simulink model "two_tanks_baseline"  (Simulink 7.3)
settings: Solver=ode45  StartTime=0.0  StopTime=1000  MaxStep=.01  RelTol=1e-3
model workspace (MAT data in the model file):
  x1o : Simulink.Parameter (value not decoded)
  a1 : Simulink.Parameter (value not decoded)
  a2 : Simulink.Parameter (value not decoded)
  A_1 : Simulink.Parameter (value not decoded)
  A_2 : Simulink.Parameter (value not decoded)
  gamma : Simulink.Parameter (value not decoded)
  g : Simulink.Parameter (value not decoded)
  x1_max : Simulink.Parameter (value not decoded)
  x2_max : Simulink.Parameter (value not decoded)
  u_max : Simulink.Parameter (value not decoded)
settings Model: Creator=Administrator  LastModifiedBy=Administrator

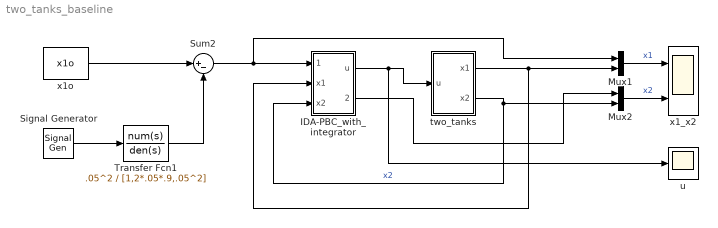
== system two_tanks_baseline ==
  IDA-PBC_with_integrator : Subsystem  mask{eps2=4, eps3=.75, q=10, A_1=A_1, A_2=A_2, a1=a1, a2=a2, gamma=gamma, u_max=u_max, x1_max=x1_max, g=g}
      mask prompts: eps2 "eps2 > 1"; eps3 "0 < eps3 < 1"; q "q > 0"; A_1 "A_1 (cm^2)"; A_2 "A_2 (cm^2)"; a1 "a1 (cm^2)"; a2 "a2 (cm^2)"; g "g (cm/s^2)"
      mask init:
      | k1 = 1;
      | if eps2 <= 1
      |     eps2 = 1.01;
      | end
      | k2 = eps2*A_2 / (4*A_1) ;
      | if eps3 >= 1
      |     eps3 = 0.99;
      | end
      | k3 = eps3*((4*k2*A_1-A_2)/(k2*A_1^2));
      | E_Qd=eig([-1/(k1*A_1),1/(k2*A_1),0;0,-1/(k2*A_2),0;k3/k1,0,-k3/k1])
      | p = [k1;-k2*gamma+k1*k2*k3-k2*k3+k2;k1^2]
      | cl_num = k2^2*gamma^2 + ((1-k1)*k2^2*k3 - 2*k2^2)*gamma + (k1-1)*k2^2*k3 + k2^2 + k1^3 + k1^2;
      | cl_den = k2^2*gamma^2 + 2*((1-k1)*k3-1)*k2^2*gamma + (k1^2-2*k1+1)*k2^2*k3^2 + 2*(k1-1)*k2^2*k3 + k2^2 + k1^4 + k1^2;
      | cl = -cl_num/cl_den
  Mux1 : Mux  Inputs=2
  Mux2 : Mux  Inputs=2
  Signal Generator : SignalGenerator  WaveForm=square  Amplitude=.95*x1o  Frequency=1/1000
  Sum2 : Sum  Inputs=|+-  OutDataType=fixdt(1, 16)  OutScaling=2^0
  Transfer Fcn1 : TransferFcn  Numerator=.05^2  Denominator=[1,2*.05*.9,.05^2]
  two_tanks : Subsystem  mask{x1o=x1o, x2o=x1o*((1-gamma)*a1/a2)^2, a1=a1, a2=a2, A_1=A_1, A_2=A_2, gamma=gamma, u_max=u_max, x1_max=x1_max, x2_max=x2_max, g=g, ku=1}
      mask prompts: x1o "x1o (cm)"; x2o "x2o (cm)"; a1 "a1 (cm2)"; a2 "a2 (cm2)"; A_1 "A_1 (cm2)"; A_2 "A_2 (cm2)"; gamma "gamma in [0,1]"; g "g (cm/s2)"
  u : Scope
      settings: YMin=5  YMax=70  SaveName=ScopeData2  SampleInput=on  SampleTime=.5
  x1_x2 : Scope  NumInputPorts=2
      settings: YMin=0~0  YMax=40~80  SampleInput=on  SampleTime=.5
  x1o : Constant  Value=x1o  OutDataType=fixdt(1, 16)  OutScaling=2^0
  wires:
  x1o/1 -> Sum2/1
  Mux1/1 -> x1_x2/1  "x1"
  two_tanks/2(x2) -> IDA-PBC_with_integrator/3(x2), Mux2/2  "x2"
  Signal Generator/1 -> Transfer Fcn1/1
  IDA-PBC_with_integrator/1(u) -> two_tanks/1(u), u/1
  Transfer Fcn1/1 -> Sum2/2
  Sum2/1 -> IDA-PBC_with_integrator/1(x1d), Mux1/1
  two_tanks/1(x1) -> IDA-PBC_with_integrator/2(x1), Mux1/2
  Mux2/1 -> x1_x2/2  "x2"
  IDA-PBC_with_integrator/2(x2d) -> Mux2/1

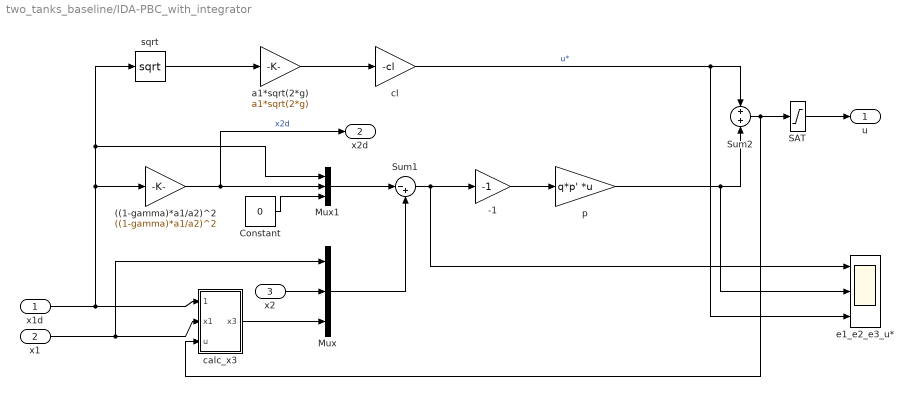
== system two_tanks_baseline/IDA-PBC_with_integrator ==
  x1d : Inport
  x1 : Inport  Port=2
  x2 : Inport  Port=3
  ((1-gamma)*a1/a2)^2 : Gain  Gain=((1-gamma)*a1/a2)^2  ParameterDataType=fixdt(1, 16)  ParameterScaling=2^0  OutDataType=fixdt(1, 16)  OutScaling=2^0
  -1 : Gain  Gain=-1  ParameterDataType=fixdt(1, 16)  ParameterScaling=2^0  OutDataType=fixdt(1, 16)  OutScaling=2^0
  Constant : Constant  Value=0  OutDataType=fixdt(1, 16)  OutScaling=2^0
  Mux : Mux  Inputs=3
  Mux1 : Mux  Inputs=3
  SAT : Saturate  UpperLimit=u_max  LowerLimit=0  OutDataType=fixdt(1, 16)  OutScaling=2^0
  Sum1 : Sum  Inputs=|-+  OutDataType=fixdt(1, 16)  OutScaling=2^0
  Sum2 : Sum  OutDataType=fixdt(1, 16)  OutScaling=2^0
  a1*sqrt(2*g) : Gain  Gain=a1*sqrt(2*g)  ParameterDataType=fixdt(1, 16)  ParameterScaling=2^0  OutDataType=fixdt(1, 16)  OutScaling=2^0
  calc_x3 : Subsystem
  cl : Gain  Gain=-cl  ParameterDataType=fixdt(1, 16)  ParameterScaling=2^0  OutDataType=fixdt(1, 16)  OutScaling=2^0
  e1_e2_e3_u* : Scope  NumInputPorts=3
      settings: YMin=-6~-50~20  YMax=3~20~55  SampleInput=on  SampleTime=.2
  p : Gain  Gain=q*p'  Multiplication=Matrix(K*u)  ParameterDataType=fixdt(1, 16)  ParameterScaling=2^0  OutDataType=fixdt(1, 16)  OutScaling=2^0
  sqrt : Math  Operator=sqrt  OutDataType=fixdt(1, 16)  OutScaling=2^0  SaturateOnIntegerOverflow=on
  u : Outport
  x2d : Outport  Port=2
  wires:
  x1d/1 -> calc_x3/1(x1d), sqrt/1, Mux1/1, ((1-gamma)*a1/a2)^2/1
  SAT/1 -> u/1
  sqrt/1 -> a1*sqrt(2*g)/1
  cl/1 -> Sum2/1, e1_e2_e3_u*/3  "u*"
  Sum2/1 -> SAT/1, calc_x3/3(u)
  x1/1 -> calc_x3/2(x1), Mux/1
  Mux1/1 -> Sum1/1
  Mux/1 -> Sum1/2
  Sum1/1 -> -1/1, e1_e2_e3_u*/1
  -1/1 -> p/1
  p/1 -> Sum2/2, e1_e2_e3_u*/2
  a1*sqrt(2*g)/1 -> cl/1
  Constant/1 -> Mux1/3
  ((1-gamma)*a1/a2)^2/1 -> Mux1/2, x2d/1  "x2d"
  calc_x3/1(x3) -> Mux/3
  x2/1 -> Mux/2

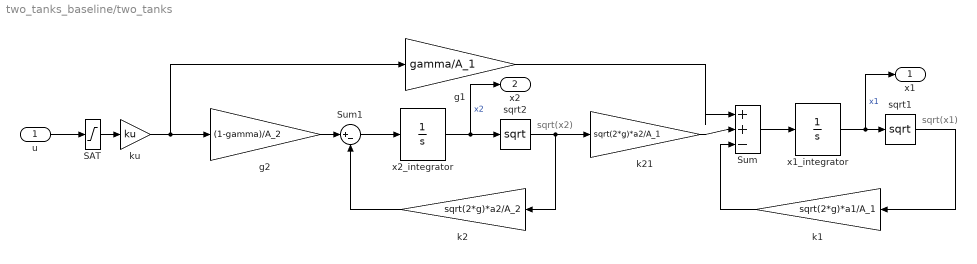
== system two_tanks_baseline/two_tanks ==
  note: sqrt(x1)
  note: sqrt(x2)
  u : Inport  OutDataType=fixdt(1, 16)  OutScaling=2^0
  SAT : Saturate  UpperLimit=u_max  LowerLimit=0  OutDataType=fixdt(1, 16)  OutScaling=2^0
  Sum : Sum  Inputs=|++-  OutDataType=fixdt(1, 16)  OutScaling=2^0
  Sum1 : Sum  Inputs=|+-  OutDataType=fixdt(1, 16)  OutScaling=2^0
  g1 : Gain  Gain=gamma/A_1  ParameterDataType=fixdt(1, 16)  ParameterScaling=2^0  OutDataType=fixdt(1, 16)  OutScaling=2^0
  g2 : Gain  Gain=(1-gamma)/A_2  ParameterDataType=fixdt(1, 16)  ParameterScaling=2^0  OutDataType=fixdt(1, 16)  OutScaling=2^0
  k1 : Gain  Gain=sqrt(2*g)*a1/A_1  ParameterDataType=fixdt(1, 16)  ParameterScaling=2^0  OutDataType=fixdt(1, 16)  OutScaling=2^0
  k2 : Gain  Gain=sqrt(2*g)*a2/A_2  ParameterDataType=fixdt(1, 16)  ParameterScaling=2^0  OutDataType=fixdt(1, 16)  OutScaling=2^0
  k21 : Gain  Gain=sqrt(2*g)*a2/A_1  ParameterDataType=fixdt(1, 16)  ParameterScaling=2^0  OutDataType=fixdt(1, 16)  OutScaling=2^0
  ku : Gain  Gain=ku  ParameterDataType=fixdt(1, 16)  ParameterScaling=2^0  OutDataType=fixdt(1, 16)  OutScaling=2^0
  sqrt1 : Math  Operator=sqrt  OutDataType=fixdt(1, 16)  OutScaling=2^0  SaturateOnIntegerOverflow=on
  sqrt2 : Math  Operator=sqrt  OutDataType=fixdt(1, 16)  OutScaling=2^0  SaturateOnIntegerOverflow=on
  x1_integrator : Integrator  InitialCondition=x1o  LimitOutput=on  UpperSaturationLimit=x1_max  LowerSaturationLimit=0
  x2_integrator : Integrator  InitialCondition=x2o  LimitOutput=on  UpperSaturationLimit=x2_max  LowerSaturationLimit=0
  x1 : Outport  OutDataType=fixdt(1, 16)  OutScaling=2^0
  x2 : Outport  Port=2  OutDataType=fixdt(1, 16)  OutScaling=2^0
  wires:
  Sum/1 -> x1_integrator/1
  k1/1 -> Sum/3
  sqrt1/1 -> k1/1
  sqrt2/1 -> k2/1, k21/1
  x2_integrator/1 -> sqrt2/1, x2/1  "x2"
  k2/1 -> Sum1/2
  Sum1/1 -> x2_integrator/1
  k21/1 -> Sum/2
  g2/1 -> Sum1/1
  x1_integrator/1 -> sqrt1/1, x1/1  "x1"
  u/1 -> SAT/1
  g1/1 -> Sum/1
  SAT/1 -> ku/1
  ku/1 -> g2/1, g1/1

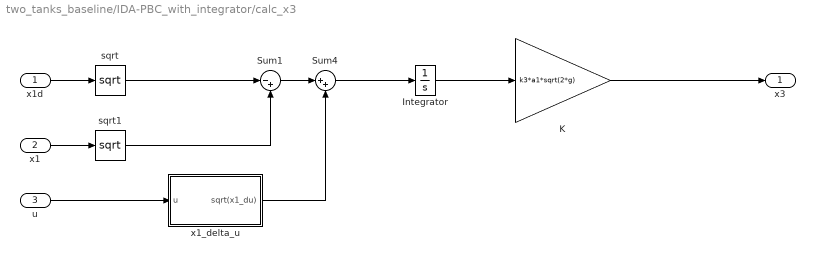
== system two_tanks_baseline/IDA-PBC_with_integrator/calc_x3 ==
  x1d : Inport
  x1 : Inport  Port=2
  u : Inport  Port=3
  Integrator : Integrator  UpperSaturationLimit=x1_max  LowerSaturationLimit=-x1_max
  K : Gain  Gain=k3*a1*sqrt(2*g)  ParameterDataType=fixdt(1, 16)  ParameterScaling=2^0  OutDataType=fixdt(1, 16)  OutScaling=2^0
  Sum1 : Sum  Inputs=|-+  OutDataType=fixdt(1, 16)  OutScaling=2^0
  Sum4 : Sum  Inputs=|++  OutDataType=fixdt(1, 16)  OutScaling=2^0
  sqrt : Math  Operator=sqrt  OutDataType=fixdt(1, 16)  OutScaling=2^0  SaturateOnIntegerOverflow=on
  sqrt1 : Math  Operator=sqrt  OutDataType=fixdt(1, 16)  OutScaling=2^0  SaturateOnIntegerOverflow=on
  x1_delta_u : Subsystem
  x3 : Outport
  wires:
  x1/1 -> sqrt1/1
  x1d/1 -> sqrt/1
  sqrt1/1 -> Sum1/2
  sqrt/1 -> Sum1/1
  Integrator/1 -> K/1
  K/1 -> x3/1
  Sum1/1 -> Sum4/1
  Sum4/1 -> Integrator/1
  x1_delta_u/1(sqrt(x1_du)) -> Sum4/2
  u/1 -> x1_delta_u/1(u)

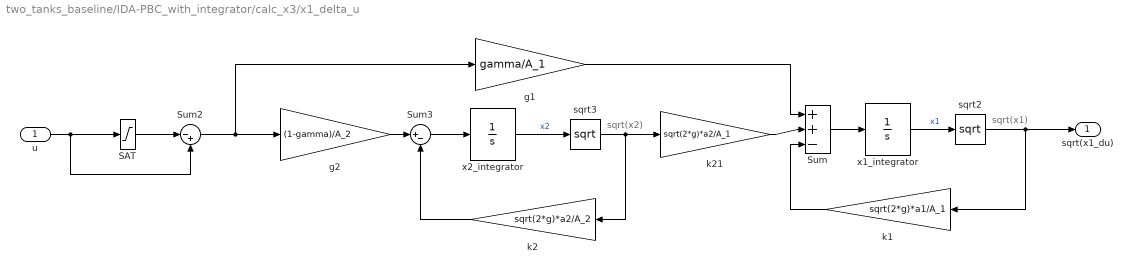
== system two_tanks_baseline/IDA-PBC_with_integrator/calc_x3/x1_delta_u ==
  note: sqrt(x1)
  note: sqrt(x2)
  u : Inport
  SAT : Saturate  UpperLimit=u_max  LowerLimit=0  OutDataType=fixdt(1, 16)  OutScaling=2^0
  Sum : Sum  Inputs=|++-  OutDataType=fixdt(1, 16)  OutScaling=2^0
  Sum2 : Sum  Inputs=|-+  OutDataType=fixdt(1, 16)  OutScaling=2^0
  Sum3 : Sum  Inputs=|+-  OutDataType=fixdt(1, 16)  OutScaling=2^0
  g1 : Gain  Gain=gamma/A_1  ParameterDataType=fixdt(1, 16)  ParameterScaling=2^0  OutDataType=fixdt(1, 16)  OutScaling=2^0
  g2 : Gain  Gain=(1-gamma)/A_2  ParameterDataType=fixdt(1, 16)  ParameterScaling=2^0  OutDataType=fixdt(1, 16)  OutScaling=2^0
  k1 : Gain  Gain=sqrt(2*g)*a1/A_1  ParameterDataType=fixdt(1, 16)  ParameterScaling=2^0  OutDataType=fixdt(1, 16)  OutScaling=2^0
  k2 : Gain  Gain=sqrt(2*g)*a2/A_2  ParameterDataType=fixdt(1, 16)  ParameterScaling=2^0  OutDataType=fixdt(1, 16)  OutScaling=2^0
  k21 : Gain  Gain=sqrt(2*g)*a2/A_1  ParameterDataType=fixdt(1, 16)  ParameterScaling=2^0  OutDataType=fixdt(1, 16)  OutScaling=2^0
  sqrt2 : Math  Operator=sqrt  OutDataType=fixdt(1, 16)  OutScaling=2^0  SaturateOnIntegerOverflow=on
  sqrt3 : Math  Operator=sqrt  OutDataType=fixdt(1, 16)  OutScaling=2^0  SaturateOnIntegerOverflow=on
  x1_integrator : Integrator  LimitOutput=on  UpperSaturationLimit=x1_max  LowerSaturationLimit=0
  x2_integrator : Integrator  LimitOutput=on  UpperSaturationLimit=x2_max  LowerSaturationLimit=0
  sqrt(x1_du) : Outport
  wires:
  u/1 -> SAT/1, Sum2/2
  SAT/1 -> Sum2/1
  Sum/1 -> x1_integrator/1
  k1/1 -> Sum/3
  sqrt2/1 -> k1/1, sqrt(x1_du)/1
  sqrt3/1 -> k2/1, k21/1
  x2_integrator/1 -> sqrt3/1  "x2"
  k2/1 -> Sum3/2
  Sum3/1 -> x2_integrator/1
  k21/1 -> Sum/2
  g2/1 -> Sum3/1
  x1_integrator/1 -> sqrt2/1  "x1"
  Sum2/1 -> g2/1, g1/1
  g1/1 -> Sum/1
